simulink model "simulink_model"  (R2021a)
settings: Solver=VariableStepAuto  StartTime=0.0  StopTime=10.0  RelTol=1e-3
libraries: simulink_extras x10, vrlib x10
settings Model: Creator=kbhar  LastModifiedBy=kbhar

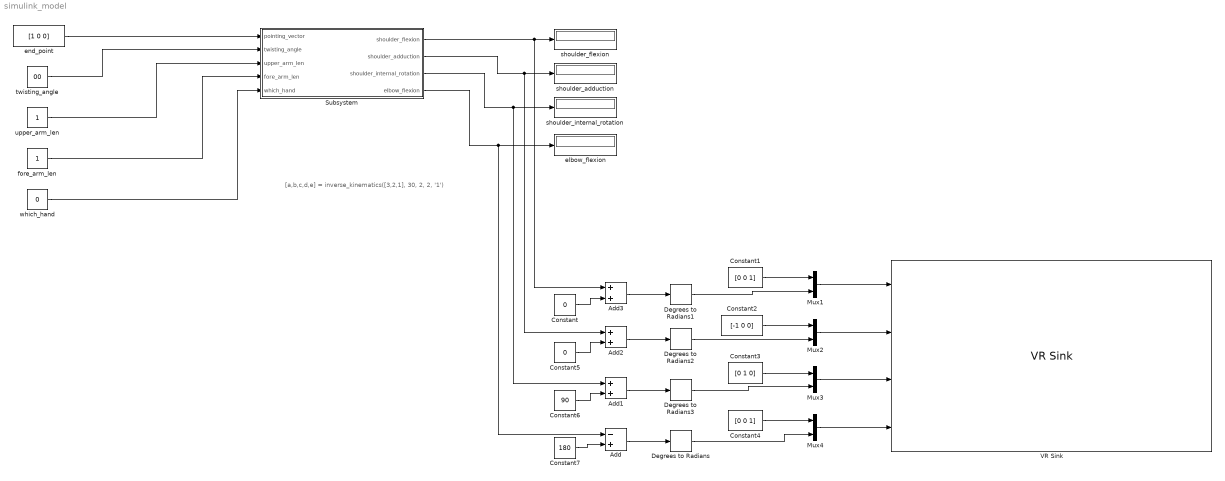
== system simulink_model ==
  note: [a,b,c,d,e] = inverse_kinematics([3,2,1], 30, 2, 2, '1')
  Add : Sum  Inputs=-+
  Add1 : Sum
  Add2 : Sum
  Add3 : Sum
  Constant : Constant  Value=0
  Constant1 : Constant  Value=[0 0 1]
  Constant2 : Constant  Value=[-1 0 0]
  Constant3 : Constant  Value=[0 1 0]
  Constant4 : Constant  Value=[0 0 1]
  Constant5 : Constant  Value=0
  Constant6 : Constant  Value=90
  Constant7 : Constant  Value=180
  Degrees to Radians{,1..3} (4 alike) : simulink_extras/Transformations/Degrees to Radians
  Mux{1..4} (4 alike) : Mux  Inputs=2
  Subsystem : Subsystem
  VR Sink : vrlib/VR Sink  InstantiateOnLoad=on  SampleTime=0.1  ViewEnable=on  RemoteChange=off  RemoteView=off  FieldsWritten=shoulderflexion.rotation.4.1.1.double#shoulderabduction.rotation.4.1.1.double#shoulderinternalrotation.rotation.4.1.1.double#elbow.rotation.4.1.1.double  WorldFileName=arm_model2.WRL  AutoView=off  VideoDimensions=[]  AllowVariableSize=off
  elbow_flexion : Display
  end_point : Constant  Value=[1 0 0]  VectorParams1D=off
  fore_arm_len : Constant
  shoulder_adduction : Display
  shoulder_flexion : Display
  shoulder_internal_rotation : Display
  twisting_angle : Constant  Value=00
  upper_arm_len : Constant
  which_hand : Constant  Value=0
  wires:
  upper_arm_len/1 -> Subsystem/3(upper_arm_len)
  fore_arm_len/1 -> Subsystem/4(fore_arm_len)
  end_point/1 -> Subsystem/1(pointing_vector)
  twisting_angle/1 -> Subsystem/2(twisting_angle)
  which_hand/1 -> Subsystem/5(which_hand)
  Subsystem/1(shoulder_flexion) -> Add3/1, shoulder_flexion/1
  Subsystem/2(shoulder_adduction) -> Add2/1, shoulder_adduction/1
  Subsystem/3(shoulder_internal_rotation) -> Add1/1, shoulder_internal_rotation/1
  Subsystem/4(elbow_flexion) -> Add/1, elbow_flexion/1
  Degrees to Radians/1 -> Mux4/2
  Degrees to Radians2/1 -> Mux2/2
  Mux4/1 -> VR Sink/4
  Mux3/1 -> VR Sink/3
  Mux2/1 -> VR Sink/2
  Mux1/1 -> VR Sink/1
  Constant1/1 -> Mux1/1
  Constant2/1 -> Mux2/1
  Constant3/1 -> Mux3/1
  Constant4/1 -> Mux4/1
  Degrees to Radians3/1 -> Mux3/2
  Degrees to Radians1/1 -> Mux1/2
  Add/1 -> Degrees to Radians/1
  Add1/1 -> Degrees to Radians3/1
  Add2/1 -> Degrees to Radians2/1
  Add3/1 -> Degrees to Radians1/1
  Constant/1 -> Add3/2
  Constant5/1 -> Add2/2
  Constant6/1 -> Add1/2
  Constant7/1 -> Add/2

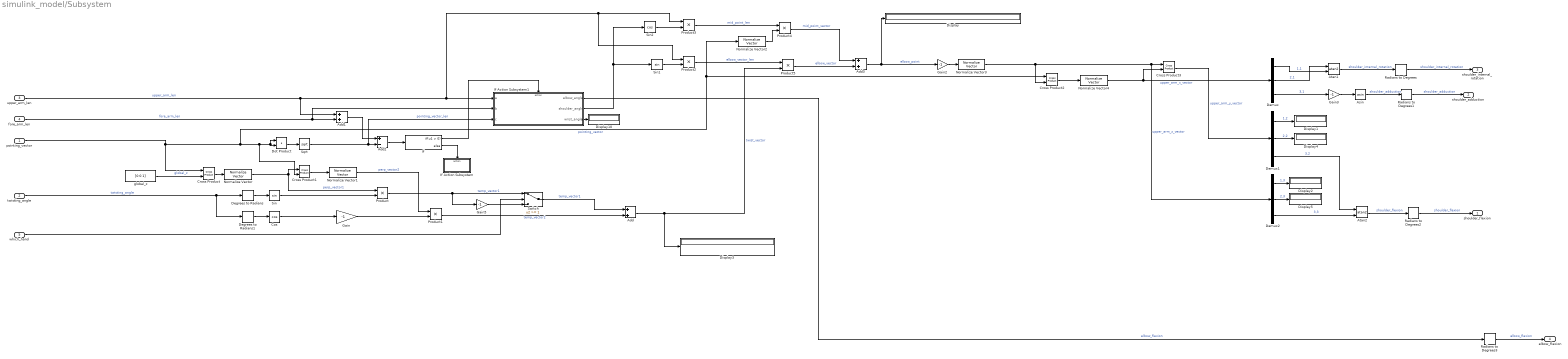
== system simulink_model/Subsystem ==
  pointing_vector : Inport
  twisting_angle : Inport  Port=2
  upper_arm_len : Inport  Port=3
  fore_arm_len : Inport  Port=4
  which_hand : Inport  Port=5
  Add : Sum
  Add1 : Sum
  Add2 : Sum  Inputs=+-
  Add3 : Sum
  Asin : Trigonometry  Operator=asin
  Atan1 : Trigonometry  Operator=atan2
  Atan2 : Trigonometry  Operator=atan2
  Cos : Trigonometry  Operator=cos
  Cross Product{,1..3} (4 alike) : vrlib/Utilities/Cross Product
  Degrees to Radians : simulink_extras/Transformations/Degrees to Radians
  Degrees to Radians1 : simulink_extras/Transformations/Degrees to Radians
  Demux : Demux  Outputs=3
  Demux1 : Demux  Outputs=3
  Demux2 : Demux  Outputs=3
  Display{,1..5,10} (7 alike) : Display
  Dot Product : DotProduct  InputSameDT=on  OutDataTypeStr=Inherit: Inherit via internal rule
  Gain{,2..3,5} (4 alike) : Gain  Gain=-1
  If : If
  If Action Subsystem : Subsystem  TreatAsAtomicUnit=on
  If Action Subsystem1 : Subsystem  TreatAsAtomicUnit=on
  Normalize Vector{,1..4} (5 alike) : vrlib/Utilities/Normalize Vector  maxzero=0
  Product{,1..5} (6 alike) : Product
  Radians to Degrees{,1..3} (4 alike) : simulink_extras/Transformations/Radians to Degrees
  Sin : Trigonometry
  Sin1 : Trigonometry
  Sin2 : Trigonometry  Operator=cos
  Sqrt : Sqrt  SaturateOnIntegerOverflow=on
  Switch : Switch  Threshold=1
  global_z : Constant  Value=[0 0 1]  VectorParams1D=off
  shoulder_flexion : Outport
  shoulder_adduction : Outport  Port=2
  shoulder_internal_rotation : Outport  Port=3
  elbow_flexion : Outport  Port=4
  wires:
  Demux1/3 -> Atan2/1  "3,2"
  global_z/1 -> Cross Product/2  "global_z"
  Cross Product/1 -> Normalize Vector/1
  Asin/1 -> Radians to Degrees1/1  "shoulder_adduction"
  Product5/1 -> Add3/2  "elbow_vector"
  Atan1/1 -> Radians to Degrees/1  "shoulder_internal_rotation"
  Cos/1 -> Gain/1
  Demux/1 -> Atan1/2  "1,1"
  Sqrt/1 -> If Action Subsystem1/3(c), Add2/2  "pointing_vector_len"
  Radians to Degrees3/1 -> elbow_flexion/1  "elbow_flexion"
  Cross Product1/1 -> Normalize Vector1/1
  Sin2/1 -> Product3/2
  Radians to Degrees2/1 -> shoulder_flexion/1  "shoulder_flexion"
  pointing_vector/1 -> Cross Product/1, Cross Product2/1, Normalize Vector2/1, Cross Product1/2, Dot Product/1, Dot Product/2  "pointing_vector"
  Cross Product2/1 -> Normalize Vector4/1
  Gain2/1 -> Normalize Vector3/1
  Normalize Vector/1 -> Cross Product1/1, Product/1  "perp_vector1"
  Product/1 -> Switch/1, Gain5/1  "temp_vector1"
  If Action Subsystem1/1(elbow_angle) -> Radians to Degrees3/1  "elbow_flexion"
  Cross Product3/1 -> Demux1/1  "upper_arm_y_vector"
  Normalize Vector1/1 -> Product1/1  "perp_vector2"
  Demux/3 -> Gain3/1  "3,1"
  Demux1/2 -> Display4/1  "2,2"
  Add1/1 -> Add2/1
  Product1/1 -> Add/2  "temp_vector2"
  fore_arm_len/1 -> If Action Subsystem1/2(b), Add1/2  "fore_arm_len"
  twisting_angle/1 -> Degrees to Radians1/1, Degrees to Radians/1  "twisting_angle"
  If/2 -> If Action Subsystem/Action
  Demux1/1 -> Display1/1  "1,2"
  Sin/1 -> Product/2
  If/1 -> If Action Subsystem1/Action
  If Action Subsystem1/2(shoulder_angle) -> Sin2/1, Sin1/1
  Gain/1 -> Product1/2
  Degrees to Radians1/1 -> Cos/1
  Degrees to Radians/1 -> Sin/1
  Sin1/1 -> Product2/2
  If Action Subsystem1/3(wrist_angle) -> Display10/1
  Demux2/2 -> Display5/1  "2,3"
  Normalize Vector3/1 -> Cross Product2/2, Demux2/1, Cross Product3/1  "upper_arm_z_vector"
  Add2/1 -> If/1
  upper_arm_len/1 -> Add1/1, Product2/1, Product3/1, If Action Subsystem1/1(a)  "upper_arm_len"
  Switch/1 -> Add/1  "temp_vector1"
  Demux2/3 -> Atan2/2  "3,3"
  Product2/1 -> Product5/1  "elbow_vector_len"
  Product4/1 -> Add3/1  "mid_point_vector"
  Add3/1 -> Gain2/1, Display/1  "elbow_point"
  Product3/1 -> Product4/1  "mid_point_len"
  Normalize Vector2/1 -> Product4/2
  Dot Product/1 -> Sqrt/1
  Demux/2 -> Atan1/1  "2,1"
  Add/1 -> Product5/2, Display3/1  "twist_vector"
  Demux2/1 -> Display2/1  "1,3"
  Normalize Vector4/1 -> Demux/1, Cross Product3/2  "upper_arm_x_vector"
  Atan2/1 -> Radians to Degrees2/1  "shoulder_flexion"
  Gain3/1 -> Asin/1
  Radians to Degrees1/1 -> shoulder_adduction/1  "shoulder_adduction"
  Radians to Degrees/1 -> shoulder_internal_rotation/1  "shoulder_internal_rotation"
  which_hand/1 -> Switch/2
  Gain5/1 -> Switch/3

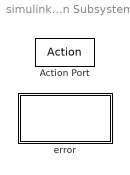
== system simulink_model/Subsystem/If Action Subsystem ==
  Action Port : ActionPort  ActionPortLabel=else
  error : MATLAB Function  TreatAsAtomicUnit=on

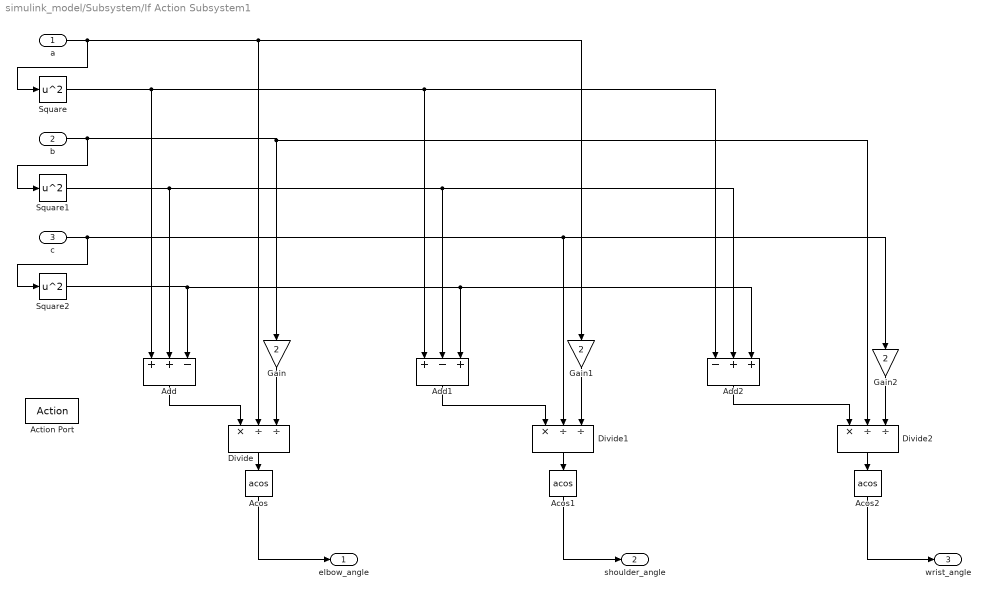
== system simulink_model/Subsystem/If Action Subsystem1 ==
  a : Inport
  b : Inport  Port=2
  c : Inport  Port=3
  Action Port : ActionPort  ActionPortLabel=if(u1 > 0)
  Acos : Trigonometry  Operator=acos
  Acos1 : Trigonometry  Operator=acos
  Acos2 : Trigonometry  Operator=acos
  Add : Sum  Inputs=++-
  Add1 : Sum  Inputs=+-+
  Add2 : Sum  Inputs=-++
  Divide : Product  Inputs=*//
  Divide1 : Product  Inputs=*//
  Divide2 : Product  Inputs=*//
  Gain : Gain  Gain=2
  Gain1 : Gain  Gain=2
  Gain2 : Gain  Gain=2
  Square : Math  Operator=square  SaturateOnIntegerOverflow=on
  Square1 : Math  Operator=square  SaturateOnIntegerOverflow=on
  Square2 : Math  Operator=square  SaturateOnIntegerOverflow=on
  elbow_angle : Outport
  shoulder_angle : Outport  Port=2
  wrist_angle : Outport  Port=3
  wires:
  a/1 -> Gain1/1, Divide/2, Square/1
  b/1 -> Divide2/2, Gain/1, Square1/1
  c/1 -> Gain2/1, Divide1/2, Square2/1
  Square/1 -> Add/1, Add1/1, Add2/1
  Square1/1 -> Add1/2, Add2/2, Add/2
  Square2/1 -> Add1/3, Add2/3, Add/3
  Add/1 -> Divide/1
  Gain/1 -> Divide/3
  Divide/1 -> Acos/1
  Acos/1 -> elbow_angle/1
  Gain1/1 -> Divide1/3
  Add1/1 -> Divide1/1
  Divide1/1 -> Acos1/1
  Acos1/1 -> shoulder_angle/1
  Add2/1 -> Divide2/1
  Gain2/1 -> Divide2/3
  Divide2/1 -> Acos2/1
  Acos2/1 -> wrist_angle/1

== matlab function simulink_model/Subsystem/If Action Subsystem/error ==
function fcn
error('not possible arm')
